simulink model "robot"  (R2018b)
settings: Solver=VariableStepAuto  StartTime=0.0  StopTime=10.0  RelTol=1e-3
values from neighbouring files (symbols this model uses):
  k_theta = 10    [robot_input.m]
  k_v = 0.1    [robot_input.m]
  L = 1    [robot_input.m]
  x_end = -10    [robot_input.m]
  xy_end = [x_end y_end]    [robot_input.m]
  y_end = -10    [robot_input.m]
libraries: simulink x3
settings Model: Creator=egorg  LastModifiedBy=egorg

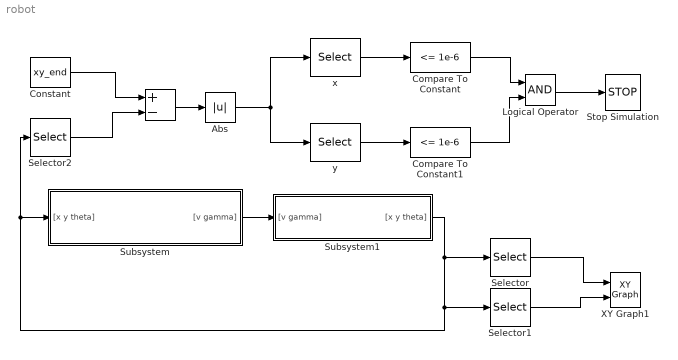
== system robot ==
  " " : Sum  Inputs=+-
  Abs : Abs
  Compare To Constant : simulink/Logic and Bit Operations/Compare To Constant  relop=<=  const=1e-6  OutDataTypeStr=boolean
  Compare To Constant1 : simulink/Logic and Bit Operations/Compare To Constant  relop=<=  const=1e-6  OutDataTypeStr=boolean
  Constant : Constant  Value=xy_end
  Logical Operator : Logic  AllPortsSameDT=off  OutDataTypeStr=boolean
  Selector : Selector  InputPortWidth=3  IndexOptions=Index vector (dialog)  Indices=1  OutputSizes=1
  Selector1 : Selector  InputPortWidth=3  IndexOptions=Index vector (dialog)  Indices=2  OutputSizes=1
  Selector2 : Selector  InputPortWidth=3  IndexOptions=Index vector (dialog)  Indices=[1 2]  OutputSizes=1
  Stop Simulation : Stop
  Subsystem : Subsystem
  Subsystem1 : Subsystem
  XY Graph1 : simulink/Sinks/XY Graph  xmin=-5  xmax=100  ymin=-5  ymax=100  st=-1
  x : Selector  InputPortWidth=2  IndexOptions=Index vector (dialog)  Indices=[1]  OutputSizes=1
  y : Selector  InputPortWidth=2  IndexOptions=Index vector (dialog)  Indices=[2]  OutputSizes=1
  wires:
  Selector2/1 -> " "/2
  Selector/1 -> XY Graph1/1
  Selector1/1 -> XY Graph1/2
  Subsystem/1("[v gamma]") -> Subsystem1/1("[v gamma]")
  Compare To Constant1/1 -> Logical Operator/2
  Compare To Constant/1 -> Logical Operator/1
  x/1 -> Compare To Constant/1
  Abs/1 -> x/1, y/1
  Subsystem1/1("[x y theta]") -> Subsystem/1("[x y theta]"), Selector2/1, Selector1/1, Selector/1
  Constant/1 -> " "/1
  Logical Operator/1 -> Stop Simulation/1
  y/1 -> Compare To Constant1/1
  " "/1 -> Abs/1

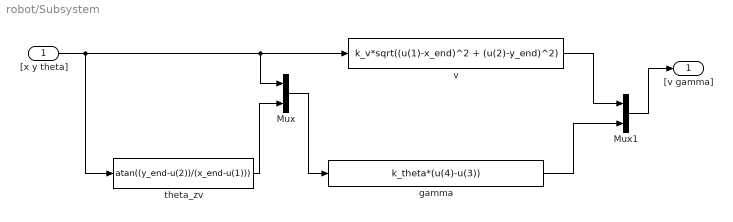
== system robot/Subsystem ==
  "[x y theta]" : Inport
  Mux : Mux  Inputs=2
  Mux1 : Mux  Inputs=2
  gamma : Fcn  Expr=k_theta*(u(4)-u(3))
  theta_zv : Fcn  Expr=atan((y_end-u(2))/(x_end-u(1)))
  v : Fcn  Expr=k_v*sqrt((u(1)-x_end)^2 + (u(2)-y_end)^2)
  "[v gamma]" : Outport
  wires:
  theta_zv/1 -> Mux/2
  "[x y theta]"/1 -> v/1, Mux/1, theta_zv/1
  Mux/1 -> gamma/1
  v/1 -> Mux1/1
  gamma/1 -> Mux1/2
  Mux1/1 -> "[v gamma]"/1

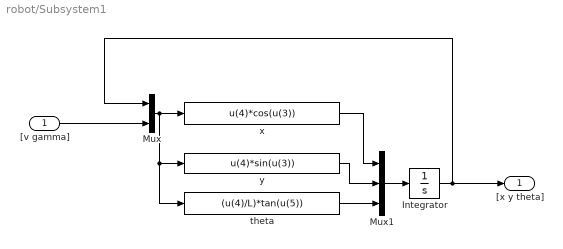
== system robot/Subsystem1 ==
  "[v gamma]" : Inport
  Integrator : Integrator
  Mux : Mux  Inputs=2
  Mux1 : Mux  Inputs=3
  theta : Fcn  Expr=(u(4)/L)*tan(u(5))
  x : Fcn  Expr=u(4)*cos(u(3))
  y : Fcn  Expr=u(4)*sin(u(3))
  "[x y theta]" : Outport
  wires:
  y/1 -> Mux1/2
  Integrator/1 -> Mux/1, "[x y theta]"/1
  theta/1 -> Mux1/3
  Mux1/1 -> Integrator/1
  "[v gamma]"/1 -> Mux/2
  x/1 -> Mux1/1
  Mux/1 -> theta/1, y/1, x/1
